simulink model "Simulation_03"  (R2014a)
settings: Solver=ode45  SolverMode=SingleTasking  StartTime=0.0  StopTime=5  FixedStep=1e-6  RelTol=1e-3
undefined symbols (not defined in the file or in its folder): sigbuilder_block
libraries: powerlib x12, simulink x2, powerlib_meascontrol x1
settings Model: CovModelRefEnable=off  Creator=Sunil Yaduvanshi  LastModifiedBy=Dell
settings SolverCC: AutoInsertRateTranBlk=on
settings DataIOCC: LimitDataPoints=off  SaveFormat=StructureWithTime
settings DebuggingCC: MergeDetectMultiDrivingBlocksExec=error  SolverPrmCheckMsg=none  FrameProcessingCompatibilityMsg=error
settings HardwareCC: ProdBitPerPointer=64  ProdLargestAtomicFloat=Float  ProdIntDivRoundTo=Zero  ProdEndianess=LittleEndian  ProdHWDeviceType=Specified
settings ModelReferenceCC: PropagateSignalLabelsOutOfModel=on

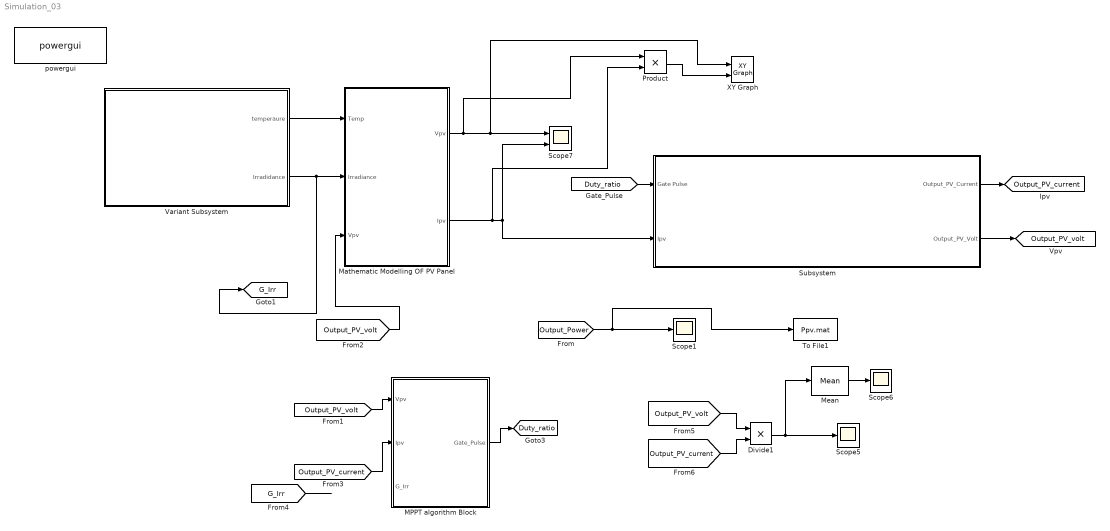
== system Simulation_03 ==
  Divide1 : Product  Inputs=**
  MPPT algorithm Block : Subsystem
  Mathematic Modelling OF PV Panel : Subsystem
      mask Display:
      | plot([0.3 0.4],[0.4 0.8]);
      | plot([0.4 0.5],[0.4 0.8]);
      | plot([0.5 0.6],[0.4 0.8]);
      | plot([0.6 0.7],[0.4 0.8]);
      | plot([0.3 0.6],[0.4 0.4]);
      | plot([0.325 0.625],[0.5 0.5]);
      | plot([0.35 0.65],[0.6 0.6]);
      | plot([0.375 0.675],[0.7 0.7]);
      | plot([0.4 0.7],[0.8 0.8]);
      | text(0.52,0.75,'PV module (V)','horizontalAlignment', 'center');
  Mean : powerlib_meascontrol/Measurements/Mean  Freq=60  Vinit=0  Ts=0
  Product : Product
  Scope1 : Scope
      settings: TimeRange=2  YMin=249.7  YMax=251.7  SaveName=ScopeData2
  Scope5 : Scope
      settings: TimeRange=0.8  YMin=222.5  YMax=262.5  SaveName=ScopeData6
  Scope6 : Scope
      settings: TimeRange=0.8  YMin=258.52  YMax=258.65  SaveName=ScopeData7
  Scope7 : Scope  NumInputPorts=2
      settings: YMin=34.5~6.825  YMax=37.5~7.275
  Subsystem : Subsystem
  To File1 : ToFile  Filename=Ppv.mat  SaveFormat=Timeseries
  Variant Subsystem : Subsystem  Variant=on
  XY Graph : simulink/Sinks/XY Graph  xmin=0  xmax=45  ymin=0  ymax=260  st=-1
  powergui : powerlib/powergui  Priority=1  SimulationMode=Discrete  SolverType=Tustin  SampleTime=1e-6  frequency=60  SPID=off  DisableSnubberDevices=off  DisableRonSwitches=off  DisableVfSwitches=off  SwTol=0  Interpol=off  DisplayEquations=off  Ts=0  methode=off  frequencyindice=0  Pbase=100e6  ErrMax=1e-4  Iterations=50  UnitsV=kV  UnitsW=MW  FunctionMessages=off  echomessages=off  HookPort=off  EnableUseOfTLC=off  x0status=blocks  RestoreLinks=warning  ResistiveCurrentMeasurement=off  Frange=[0:2:500]  Ylog=off  Xlog=on  ShowGrid=off  save=off  variable=ZData  structure=0  ZoomFFT=off  StartTime=0.0  cycles=1  DisplayStyle=1  fundamental=60  FreqAxis=off  MaxFrequency=1000  frequencyindicesteady=1  RmsSteady=1  display=off
  tag scope: Duty_ratio=global, G_Irr=global, Output_PV_current=global, Output_PV_volt=global
  wires:
  [Output_Power] -> To File1/1, Scope1/1
  [Output_PV_volt] -> Divide1/1
  [Output_PV_current] -> Divide1/2
  Divide1/1 -> Scope5/1, Mean/1
  Mean/1 -> Scope6/1
  Variant Subsystem/1(temperaure) -> Mathematic Modelling OF PV Panel/1(Temp)
  Variant Subsystem/2("Irradidance ") -> [G_Irr], Mathematic Modelling OF PV Panel/2(Irradiance)
  Mathematic Modelling OF PV Panel/2(Ipv) -> Product/2, Subsystem/2(Ipv), Scope7/2
  [Output_PV_volt] -> Mathematic Modelling OF PV Panel/3(Vpv)
  [Duty_ratio] -> Subsystem/1(Gate Pulse)
  Subsystem/1(Output_PV_Current) -> [Output_PV_current]
  Subsystem/2(Output_PV_Volt) -> [Output_PV_volt]
  [Output_PV_volt] -> MPPT algorithm Block/1(Vpv)
  [Output_PV_current] -> MPPT algorithm Block/2(Ipv)
  MPPT algorithm Block/1("Gate_Pulse ") -> [Duty_ratio]
  [G_Irr] -> ?
  Mathematic Modelling OF PV Panel/1("Vpv ") -> Product/1, XY Graph/1, Scope7/1
  Product/1 -> XY Graph/2

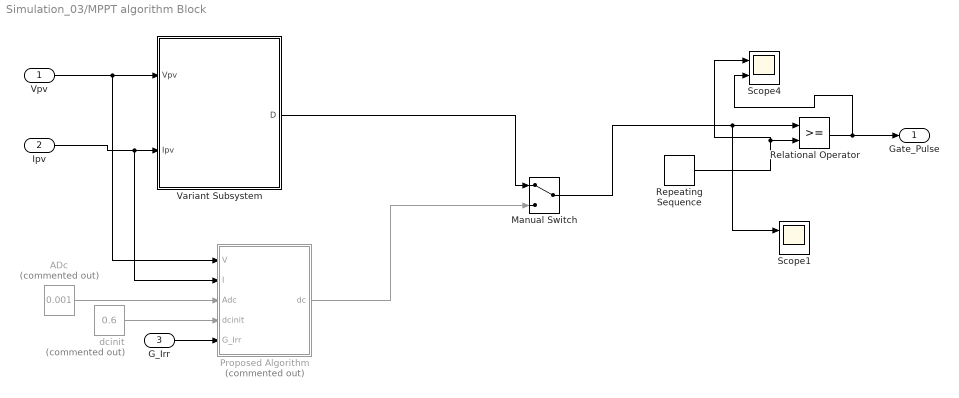
== system Simulation_03/MPPT algorithm Block ==
  Vpv : Inport
  Ipv : Inport  Port=2
  G_Irr : Inport  Port=3
  "ADc\t" : Constant  Commented=on  Value=0.001
  Manual Switch : ManualSwitch
  Proposed Algorithm : MATLAB Function  Commented=on  TreatAsAtomicUnit=on
  Relational Operator : RelationalOperator  OutDataTypeStr=boolean
  Repeating Sequence : simulink/Sources/Repeating Sequence  rep_seq_t=[0 1/40000 1/20000]  rep_seq_y=[0 1 0]
  Scope1 : Scope  NumInputPorts=2
      settings: YMin=2.6~0  YMax=2.9~1
  Scope4 : Scope  NumInputPorts=2
      settings: YMin=0~0  YMax=1~1  SaveName=ScopeData5
  Variant Subsystem : Subsystem  Variant=on
  dcinit : Constant  Commented=on  Value=0.6
  "Gate_Pulse " : Outport
  wires:
  Relational Operator/1 -> "Gate_Pulse "/1, Scope4/2
  Repeating Sequence/1 -> Scope4/1, Relational Operator/2
  Ipv/1 -> Proposed Algorithm/2(I), Variant Subsystem/2(Ipv)
  Vpv/1 -> Proposed Algorithm/1(V), Variant Subsystem/1(Vpv)
  Manual Switch/1 -> Scope1/1, Relational Operator/1
  Variant Subsystem/1(D) -> Manual Switch/1
  dcinit/1 -> Proposed Algorithm/4(dcinit)
  "ADc\t"/1 -> Proposed Algorithm/3(Adc)
  Proposed Algorithm/1(dc) -> Manual Switch/2
  G_Irr/1 -> Proposed Algorithm/5(G_Irr)

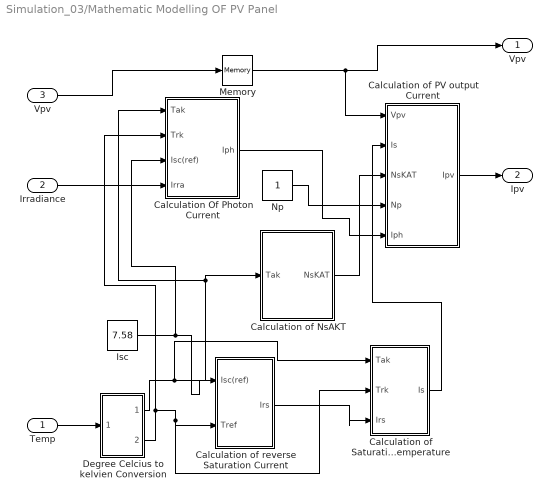
== system Simulation_03/Mathematic Modelling OF PV Panel ==
  Temp : Inport
  Irradiance : Inport  Port=2
  Vpv : Inport  Port=3
  "Calculation Of Photon Current " : Subsystem
  Calculation of Saturation Current Varies With Temperature : Subsystem
  Calculation of NsAKT : Subsystem
  "Calculation of PV output Current " : Subsystem
  Calculation of reverse Saturation Current : Subsystem
  Degree Celcius to kelvien Conversion : Subsystem
  Isc : Constant  Value=7.58
  Memory : Memory
  Np : Constant
  "Vpv " : Outport
  Ipv : Outport  Port=2
  wires:
  Calculation of Saturation Current Varies With Temperature/1(Is) -> "Calculation of PV output Current "/2(Is)
  Calculation of reverse Saturation Current/1(Irs) -> Calculation of Saturation Current Varies With Temperature/3("Irs ")
  Np/1 -> "Calculation of PV output Current "/4(Np)
  Temp/1 -> Degree Celcius to kelvien Conversion/1("Top ")
  "Calculation of PV output Current "/1("Ipv ") -> Ipv/1
  Irradiance/1 -> "Calculation Of Photon Current "/4(Irra)
  Degree Celcius to kelvien Conversion/1(Tak) -> Calculation of Saturation Current Varies With Temperature/1(Tak), "Calculation Of Photon Current "/1(Tak), Calculation of NsAKT/1("Tak ")
  "Calculation Of Photon Current "/1(Iph) -> "Calculation of PV output Current "/5(Iph)
  Calculation of NsAKT/1(NsKAT) -> "Calculation of PV output Current "/3(NsKAT)
  Isc/1 -> "Calculation Of Photon Current "/3(Isc(ref)), Calculation of reverse Saturation Current/1("Isc(ref) ")
  Degree Celcius to kelvien Conversion/2(Trk) -> "Calculation Of Photon Current "/2(Trk), Calculation of Saturation Current Varies With Temperature/2("Trk "), Calculation of reverse Saturation Current/2("Tref ")
  Vpv/1 -> Memory/1
  Memory/1 -> "Calculation of PV output Current "/1(Vpv), "Vpv "/1

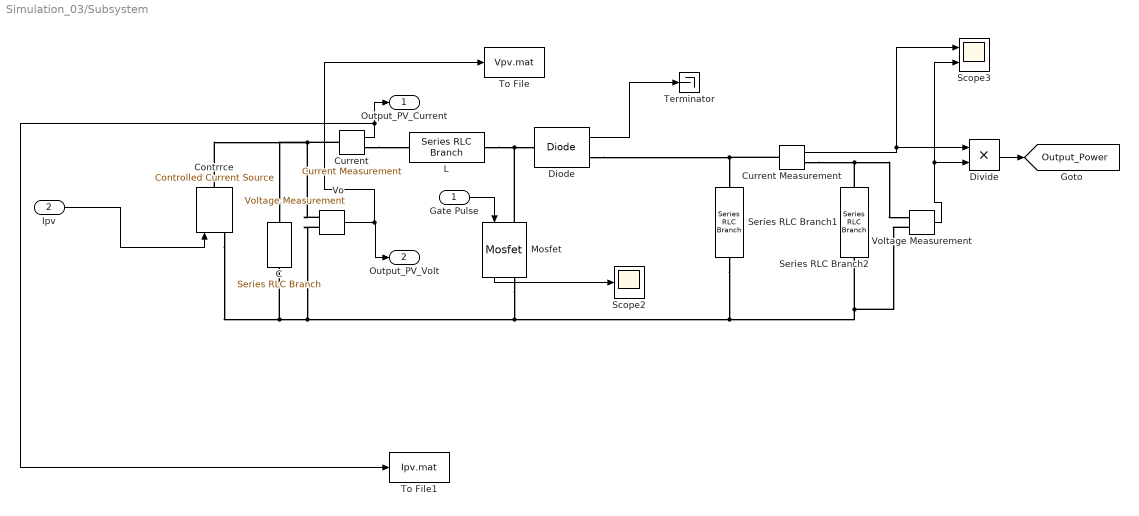
== system Simulation_03/Subsystem ==
  Gate Pulse : Inport
  Ipv : Inport  Port=2
  C : powerlib/Elements/Series RLC Branch  LConnTagsString=__new0  RConnTagsString=__new0  BranchType=C  Resistance=10  Inductance=5e-3  SetiL0=on  InitialCurrent=0  Capacitance=1e-6  Setx0=off  InitialVoltage=0  Measurements=None
  Contrrce : powerlib/Electrical Sources/Controlled Current Source  Initialize=on  Source_Type=DC  Amplitude=0  Phase=0  Frequency=0  Measurements=None
  "Current " : powerlib/Measurements/Current Measurement  PhasorSimulation=off  OutputType=Complex  PSBequivalent=0
  Current Measurement : powerlib/Measurements/Current Measurement  PhasorSimulation=off  OutputType=Complex  PSBequivalent=0
  Diode : powerlib/Power Electronics/Diode  Ron=0.001  Lon=0  Vf=0.8  IC=0  UseSnubber=off  Rs=500*0  Cs=250e-9*0  Measurements=on
  Divide : Product  Inputs=**
  L : powerlib/Elements/Series RLC Branch  LConnTagsString=__new0  RConnTagsString=__new0  BranchType=L  Resistance=10  Inductance=5e-3  SetiL0=on  InitialCurrent=0  Capacitance=1e-6  Setx0=off  InitialVoltage=0  Measurements=None
  Mosfet : powerlib/Power Electronics/Mosfet  Ron=0.1  Lon=0  Rd=0.01  Vfd=0  IC=0  Rs=1e5  Cs=inf  Measurements=on
  Scope2 : Scope
      settings: YMin=-5.49725  YMax=49.47525  SaveName=ScopeData3
  Scope3 : Scope  NumInputPorts=2
      settings: YMin=2.52~100.8  YMax=2.536~101.45  SaveName=ScopeData4
  Series RLC Branch1 : powerlib/Elements/Series RLC Branch  LConnTagsString=__new0  RConnTagsString=__new0  BranchType=C  Resistance=1  Inductance=5e-3  SetiL0=on  InitialCurrent=0  Capacitance=270e-6  Setx0=on  InitialVoltage=0  Measurements=None
  Series RLC Branch2 : powerlib/Elements/Series RLC Branch  LConnTagsString=__new0  RConnTagsString=__new0  BranchType=R  Resistance=60  Inductance=5e-3  SetiL0=on  InitialCurrent=0  Capacitance=1e-6  Setx0=off  InitialVoltage=0  Measurements=None
  Terminator : Terminator
  To File : ToFile  Filename=Vpv.mat  SaveFormat=Timeseries
  To File1 : ToFile  Filename=Ipv.mat  SaveFormat=Timeseries
  Vo : powerlib/Measurements/Voltage Measurement  PhasorSimulation=off  OutputType=Complex  PSBequivalent=0
  Voltage Measurement : powerlib/Measurements/Voltage Measurement  PhasorSimulation=off  OutputType=Complex  PSBequivalent=0
  Output_PV_Current : Outport
  Output_PV_Volt : Outport  Port=2
  tag scope: Output_Power=global
  wires:
  Ipv/1 -> Contrrce/1
  Diode/1 -> Terminator/1
  Divide/1 -> [Output_Power]
  Voltage Measurement/1 -> Scope3/2, Divide/2
  Vo/1 -> To File/1, Output_PV_Volt/1
  Gate Pulse/1 -> Mosfet/1
  "Current "/1 -> To File1/1, Output_PV_Current/1
  Current Measurement/1 -> Divide/1, Scope3/1
  Mosfet/1 -> Scope2/1
  connections:
  Diode/RConn1 -- Current Measurement/LConn1 -- Series RLC Branch1/LConn1
  Vo/LConn1 -- Contrrce/RConn1 -- C/LConn1 -- "Current "/LConn1
  Series RLC Branch2/LConn1 -- Current Measurement/RConn1 -- Voltage Measurement/LConn1
  Contrrce/LConn1 -- C/RConn1 -- Vo/LConn2 -- Mosfet/RConn1 -- Series RLC Branch1/RConn1 -- Voltage Measurement/LConn2 -- Series RLC Branch2/RConn1
  "Current "/RConn1 -- L/LConn1
  L/RConn1 -- Mosfet/LConn1 -- Diode/LConn1

== system Simulation_03/Variant Subsystem ==
  note: 1) Only subsystems can be added as variant choices at this level
      | 2) Blocks cannot be connected at this level as connectivity is
      | automatically determined at simulation, based on the active variant
  Irradiance Variatioin : Subsystem  TreatAsAtomicUnit=on  VariantControl=Irradiance
  "Temperature Variation " : Subsystem  TreatAsAtomicUnit=on  VariantControl=Temperature
  temperaure : Outport
  "Irradidance " : Outport  Port=2

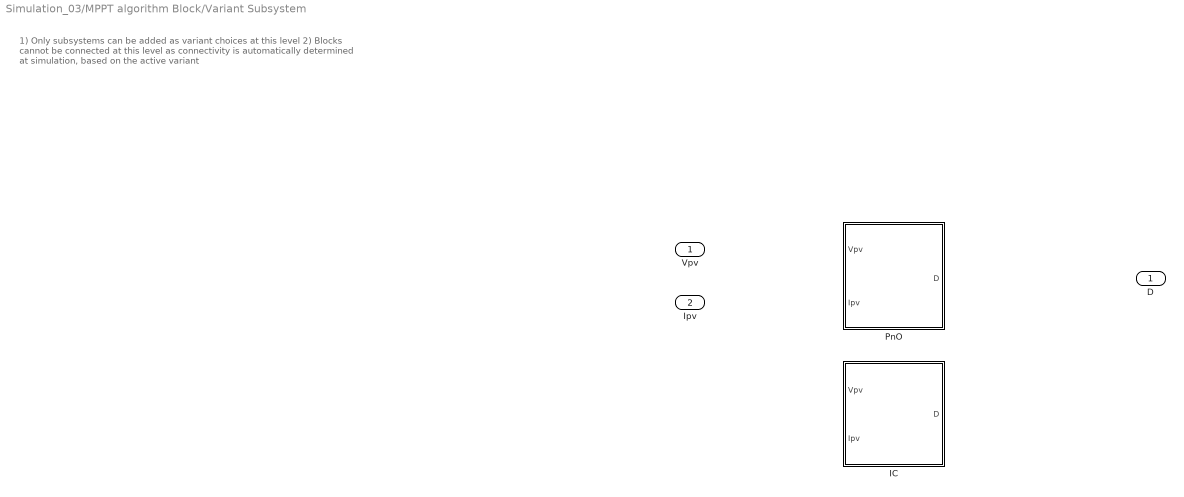
== system Simulation_03/MPPT algorithm Block/Variant Subsystem ==
  note: 1) Only subsystems can be added as variant choices at this level
      | 2) Blocks cannot be connected at this level as connectivity is
      | automatically determined at simulation, based on the active variant
  Vpv : Inport
  Ipv : Inport  Port=2
  IC : Subsystem  TreatAsAtomicUnit=on  VariantControl=IC
  PnO : Subsystem  TreatAsAtomicUnit=on  VariantControl=PnO
  D : Outport

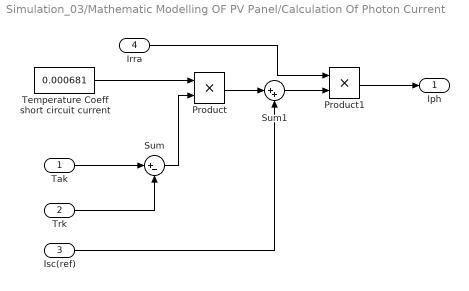
== system Simulation_03/Mathematic Modelling OF PV Panel/Calculation Of Photon Current  ==
  Tak : Inport
  Trk : Inport  Port=2
  Isc(ref) : Inport  Port=3
  Irra : Inport  Port=4
  Product : Product
  Product1 : Product
  Sum : Sum  Inputs=|+-
  Sum1 : Sum  Inputs=|++
  "Temperature Coeff short circuit current " : Constant  Value=0.000681
  Iph : Outport
  wires:
  Product/1 -> Sum1/1
  Trk/1 -> Sum/2
  "Temperature Coeff short circuit current "/1 -> Product/1
  Irra/1 -> Product1/1
  Isc(ref)/1 -> Sum1/2
  Tak/1 -> Sum/1
  Sum1/1 -> Product1/2
  Sum/1 -> Product/2
  Product1/1 -> Iph/1

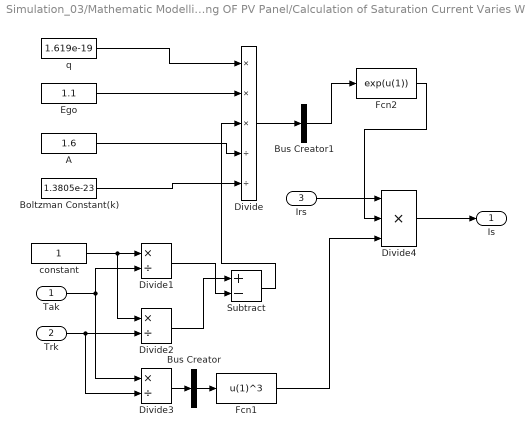
== system Simulation_03/Mathematic Modelling OF PV Panel/Calculation of Saturation Current Varies With Temperature ==
  Tak : Inport
  "Trk " : Inport  Port=2
  "Irs " : Inport  Port=3
  "A " : Constant  Value=1.6
  Boltzman Constant(k) : Constant  Value=1.3805e-23
  Bus Creator : BusCreator  Inputs=1
  Bus Creator1 : BusCreator  Inputs=1
  Divide : Product  Inputs=***//
  Divide1 : Product  Inputs=*/
  Divide2 : Product  Inputs=*/
  Divide3 : Product  Inputs=*/
  Divide4 : Product  Inputs=***
  Ego : Constant  Value=1.1
  Fcn1 : Fcn  Expr=u(1)^3
  Fcn2 : Fcn  Expr=exp(u(1))
  Subtract : Sum  Inputs=+-
  "constant " : Constant
  "q " : Constant  Value=1.619e-19
  Is : Outport
  wires:
  "constant "/1 -> Divide2/1, Divide1/1
  Bus Creator1/1 -> Fcn2/1
  Divide/1 -> Bus Creator1/1
  Divide1/1 -> Subtract/2
  Fcn1/1 -> Divide4/3
  Divide2/1 -> Subtract/1
  Tak/1 -> Divide1/2, Divide3/1
  Fcn2/1 -> Divide4/2
  "Trk "/1 -> Divide3/2, Divide2/2
  "A "/1 -> Divide/4
  Ego/1 -> Divide/2
  Subtract/1 -> Divide/3
  Boltzman Constant(k)/1 -> Divide/5
  "q "/1 -> Divide/1
  "Irs "/1 -> Divide4/1
  Divide4/1 -> Is/1
  Bus Creator/1 -> Fcn1/1
  Divide3/1 -> Bus Creator/1

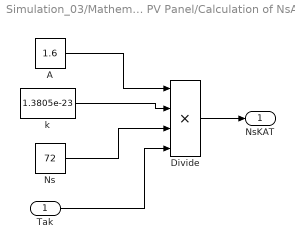
== system Simulation_03/Mathematic Modelling OF PV Panel/Calculation of NsAKT ==
  "Tak " : Inport
  A : Constant  Value=1.6
  Divide : Product  Inputs=****
  Ns : Constant  Value=72
  k : Constant  Value=1.3805e-23
  NsKAT : Outport
  wires:
  Ns/1 -> Divide/3
  A/1 -> Divide/1
  k/1 -> Divide/2
  "Tak "/1 -> Divide/4
  Divide/1 -> NsKAT/1

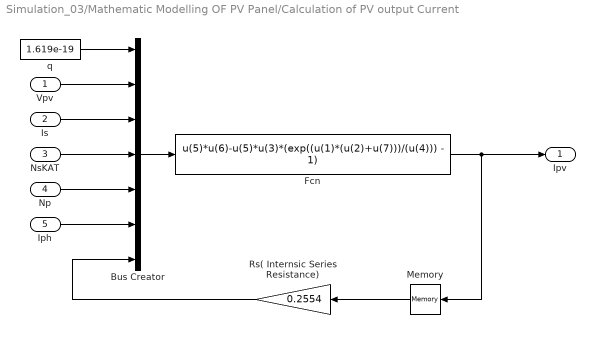
== system Simulation_03/Mathematic Modelling OF PV Panel/Calculation of PV output Current  ==
  Vpv : Inport
  Is : Inport  Port=2
  NsKAT : Inport  Port=3
  Np : Inport  Port=4
  Iph : Inport  Port=5
  Bus Creator : BusCreator  Inputs=7
  Fcn : Fcn  Expr=u(5)*u(6)-u(5)*u(3)*(exp((u(1)*(u(2)+u(7)))/(u(4))) - 1)
  Memory : Memory
  Rs( Internsic Series Resistance) : Gain  Gain=0.2554
  q : Constant  Value=1.619e-19
  "Ipv " : Outport
  wires:
  Vpv/1 -> Bus Creator/2
  Is/1 -> Bus Creator/3
  Fcn/1 -> Memory/1, "Ipv "/1
  Bus Creator/1 -> Fcn/1
  Rs( Internsic Series Resistance)/1 -> Bus Creator/7
  Iph/1 -> Bus Creator/6
  Np/1 -> Bus Creator/5
  q/1 -> Bus Creator/1
  NsKAT/1 -> Bus Creator/4
  Memory/1 -> Rs( Internsic Series Resistance)/1

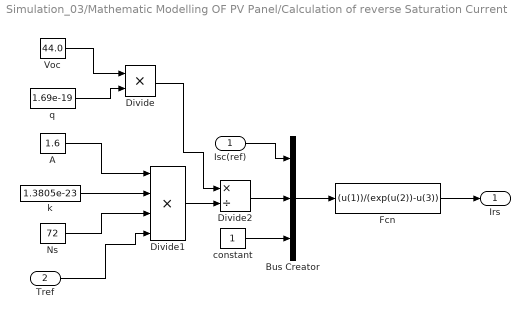
== system Simulation_03/Mathematic Modelling OF PV Panel/Calculation of reverse Saturation Current ==
  "Isc(ref) " : Inport
  "Tref " : Inport  Port=2
  A : Constant  Value=1.6
  Bus Creator : BusCreator  Inputs=3
  Divide : Product  Inputs=**
  Divide1 : Product  Inputs=****
  Divide2 : Product  Inputs=*/
  Fcn : Fcn  Expr=(u(1))/(exp(u(2))-u(3))
  Ns : Constant  Value=72
  Voc : Constant  Value=44.0
  "constant " : Constant
  k : Constant  Value=1.3805e-23
  q : Constant  Value=1.69e-19
  Irs : Outport
  wires:
  Voc/1 -> Divide/1
  Divide/1 -> Divide2/1
  k/1 -> Divide1/2
  "constant "/1 -> Bus Creator/3
  Divide2/1 -> Bus Creator/2
  Bus Creator/1 -> Fcn/1
  "Tref "/1 -> Divide1/4
  Fcn/1 -> Irs/1
  q/1 -> Divide/2
  A/1 -> Divide1/1
  "Isc(ref) "/1 -> Bus Creator/1
  Ns/1 -> Divide1/3
  Divide1/1 -> Divide2/2

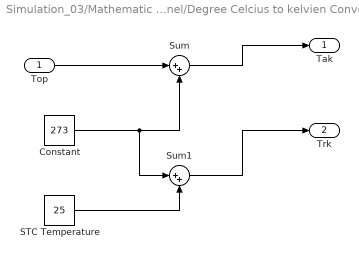
== system Simulation_03/Mathematic Modelling OF PV Panel/Degree Celcius to kelvien Conversion ==
  "Top " : Inport
  Constant : Constant  Value=273
  STC Temperature : Constant  Value=25
  Sum : Sum  Inputs=|++
  Sum1 : Sum  Inputs=|++
  Tak : Outport
  Trk : Outport  Port=2
  wires:
  Sum1/1 -> Trk/1
  Constant/1 -> Sum1/1, Sum/2
  "Top "/1 -> Sum/1
  Sum/1 -> Tak/1
  STC Temperature/1 -> Sum1/2

== system Simulation_03/Variant Subsystem/Irradiance Variatioin ==
  Insolation1 : Subsystem  Tag=STV Subsys  LoadFcn=sigbuilder_block('load');  StartFcn=sigbuilder_block('start');  StopFcn=sigbuilder_block('stop');  ClipboardFcn=sigbuilder_block('clipboard');  mask(Sigbuilder block){}
      mask help: Simulink:masks:SigbuilderBlock_MD
      mask init:
      | if ~strcmp(get_param(bdroot(gcbh),'SimulationStatus'),'stopped') tuvar = sigbuilder_block('maskInit'); end
      settings: CopyFcn=sigbuilder_block('copy');  DeleteFcn=sigbuilder_block('delete');  ModelCloseFcn=sigbuilder_block('modelClose');  PreSaveFcn=sigbuilder_block('preSave');  PauseFcn=sigbuilder_block('pause')  ContinueFcn=sigbuilder_block('continue')  NameChangeFcn=sigbuilder_block('namechange');  OpenFcn=sigbuilder_block('open',[211.5 118.5 550.5 394.5 ]);  CloseFcn=sigbuilder_block('close');
      mask Display: plot(0, 0, 100, 100,[2, 2, 32, 32, 2], [68, 8, 8, 68, 68],[32, 2], [38, 38], [32, 19, 2],[53, 60, 44], [32, 17, 17, 2],[16, 16, 31, 31]);txt = getActiveGroup(gcbh);text(2, 100, txt,'verticalAlignment', 'top');
  "Temperature " : Subsystem  Tag=STV Subsys  LoadFcn=sigbuilder_block('load');  StartFcn=sigbuilder_block('start');  StopFcn=sigbuilder_block('stop');  ClipboardFcn=sigbuilder_block('clipboard');  mask(Sigbuilder block){}
      mask help: Simulink:masks:SigbuilderBlock_MD
      mask init:
      | if ~strcmp(get_param(bdroot(gcbh),'SimulationStatus'),'stopped') tuvar = sigbuilder_block('maskInit'); end
      settings: CopyFcn=sigbuilder_block('copy');  DeleteFcn=sigbuilder_block('delete');  ModelCloseFcn=sigbuilder_block('modelClose');  PreSaveFcn=sigbuilder_block('preSave');  PauseFcn=sigbuilder_block('pause');  ContinueFcn=sigbuilder_block('continue');  NameChangeFcn=sigbuilder_block('namechange');  OpenFcn=sigbuilder_block('open',[351 -51.75 543 385.5 ]);  CloseFcn=sigbuilder_block('close');
      mask Display: plot(0, 0, 100, 100,[2, 2, 32, 32, 2], [68, 8, 8, 68, 68],[32, 2], [38, 38], [32, 19, 2],[53, 60, 44], [32, 17, 17, 2],[16, 16, 31, 31]);txt = getActiveGroup(gcbh);text(2, 100, txt,'verticalAlignment', 'top');
  temperaure : Outport
  "Irradidance " : Outport  Port=2
  wires:
  "Temperature "/1(Signal 1) -> temperaure/1
  Insolation1/1(irradiation) -> "Irradidance "/1

== system Simulation_03/Variant Subsystem/Temperature Variation  ==
  Insolation1 : Subsystem  Tag=STV Subsys  LoadFcn=sigbuilder_block('load');  StartFcn=sigbuilder_block('start');  StopFcn=sigbuilder_block('stop');  ClipboardFcn=sigbuilder_block('clipboard');  mask(Sigbuilder block){}
      mask help: Simulink:masks:SigbuilderBlock_MD
      mask init:
      | if ~strcmp(get_param(bdroot(gcbh),'SimulationStatus'),'stopped') tuvar = sigbuilder_block('maskInit'); end
      settings: CopyFcn=sigbuilder_block('copy');  DeleteFcn=sigbuilder_block('delete');  ModelCloseFcn=sigbuilder_block('modelClose');  PreSaveFcn=sigbuilder_block('preSave');  PauseFcn=sigbuilder_block('pause')  ContinueFcn=sigbuilder_block('continue')  NameChangeFcn=sigbuilder_block('namechange');  OpenFcn=sigbuilder_block('open',[557.25 17.25 550.5 394.5 ]);  CloseFcn=sigbuilder_block('close');
      mask Display: plot(0, 0, 100, 100,[2, 2, 32, 32, 2], [68, 8, 8, 68, 68],[32, 2], [38, 38], [32, 19, 2],[53, 60, 44], [32, 17, 17, 2],[16, 16, 31, 31]);txt = getActiveGroup(gcbh);text(2, 100, txt,'verticalAlignment', 'top');
  Temperature : Subsystem  Tag=STV Subsys  LoadFcn=sigbuilder_block('load');  StartFcn=sigbuilder_block('start');  StopFcn=sigbuilder_block('stop');  ClipboardFcn=sigbuilder_block('clipboard');  mask(Sigbuilder block){}
      mask help: Simulink:masks:SigbuilderBlock_MD
      mask init:
      | if ~strcmp(get_param(bdroot(gcbh),'SimulationStatus'),'stopped') tuvar = sigbuilder_block('maskInit'); end
      settings: CopyFcn=sigbuilder_block('copy');  DeleteFcn=sigbuilder_block('delete');  ModelCloseFcn=sigbuilder_block('modelClose');  PreSaveFcn=sigbuilder_block('preSave');  PauseFcn=sigbuilder_block('pause');  ContinueFcn=sigbuilder_block('continue');  NameChangeFcn=sigbuilder_block('namechange');  OpenFcn=sigbuilder_block('open',[437.25 180 550.5 395.25 ]);  CloseFcn=sigbuilder_block('close');
      mask Display: plot(0, 0, 100, 100,[2, 2, 32, 32, 2], [68, 8, 8, 68, 68],[32, 2], [38, 38], [32, 19, 2],[53, 60, 44], [32, 17, 17, 2],[16, 16, 31, 31]);txt = getActiveGroup(gcbh);text(2, 100, txt,'verticalAlignment', 'top');
  temperaure : Outport
  "Irradidance " : Outport  Port=2
  wires:
  Temperature/1(Signal 1) -> temperaure/1
  Insolation1/1(irradiation) -> "Irradidance "/1

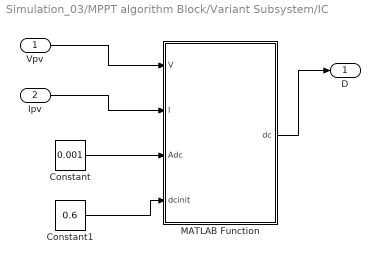
== system Simulation_03/MPPT algorithm Block/Variant Subsystem/IC ==
  Vpv : Inport  OutDataTypeStr=double  PortDimensions=1  SampleTime=[0.0001,0]
  Ipv : Inport  Port=2  OutDataTypeStr=double  PortDimensions=1  SampleTime=[0.0001,0]
  Constant : Constant  Value=0.001
  Constant1 : Constant  Value=0.6
  MATLAB Function : MATLAB Function  TreatAsAtomicUnit=on
  D : Outport  OutDataTypeStr=double  PortDimensions=1  SampleTime=[0.0001,0]
  wires:
  Vpv/1 -> MATLAB Function/1(V)
  Ipv/1 -> MATLAB Function/2(I)
  MATLAB Function/1(dc) -> D/1
  Constant1/1 -> MATLAB Function/4(dcinit)
  Constant/1 -> MATLAB Function/3(Adc)

== system Simulation_03/MPPT algorithm Block/Variant Subsystem/PnO ==
  Vpv : Inport
  Ipv : Inport  Port=2
  MATLAB Function : MATLAB Function  TreatAsAtomicUnit=on
  D : Outport
  wires:
  Ipv/1 -> MATLAB Function/2(PV_current)
  Vpv/1 -> MATLAB Function/1(PV_volt)
  MATLAB Function/1(D) -> D/1

== system Simulation_03/Variant Subsystem/Irradiance Variatioin/Insolation1 ==
  Demux : Demux  Tag=STV Demux  Outputs=1
  FromWs : FromWorkspace  Tag=STV FromWs  VariableName=tuvar  SampleTime=0
      SigBuilderData=|
      | common.afterFinalStr = 'Extrapolate'
      | common.sampleTime = 0
      | dataSet.timeRange = [0 6]
      | dataSet.name = 'Group 1'
      | sbobj.Groups.Name = 'Group 1'
      | sbobj.Groups.Signals.Name = 'irradiation'
      | sbobj.Groups.Signals.XData = [0 2 2 3.99 4 6]
      | sbobj.Groups.Signals.YData = [0.6 0.6 0.8 0.8 1 1]
  irradiation : Outport  Tag=STV Outport
  wires:
  FromWs/1 -> Demux/1
  Demux/1 -> irradiation/1

== system Simulation_03/Variant Subsystem/Irradiance Variatioin/Temperature  ==
  Demux : Demux  Tag=STV Demux  Outputs=1
  FromWs : FromWorkspace  Tag=STV FromWs  VariableName=tuvar  SampleTime=0
      SigBuilderData=|
      | common.afterFinalStr = 'Extrapolate'
      | common.sampleTime = 0
      | dataSet.timeRange = [0 10]
      | dataSet.name = 'Group 1'
      | sbobj.Groups.Name = 'Group 1'
      | sbobj.Groups.Signals.Name = 'Signal 1'
      | sbobj.Groups.Signals.XData = [0 1 2 10]
      | sbobj.Groups.Signals.YData = [25 25 25 25]
  Signal 1 : Outport  Tag=STV Outport
  wires:
  FromWs/1 -> Demux/1
  Demux/1 -> Signal 1/1

== system Simulation_03/Variant Subsystem/Temperature Variation /Insolation1 ==
  Demux : Demux  Tag=STV Demux  Outputs=1
  FromWs : FromWorkspace  Tag=STV FromWs  VariableName=tuvar  SampleTime=0
      SigBuilderData=|
      | common.afterFinalStr = 'Extrapolate'
      | common.sampleTime = 0
      | dataSet.timeRange = [0 6]
      | dataSet.name = 'Group 1'
      | sbobj.Groups.Name = 'Group 1'
      | sbobj.Groups.Signals.Name = 'irradiation'
      | sbobj.Groups.Signals.XData = [0 2 3.99 4 6]
      | sbobj.Groups.Signals.YData = [1 1 1 1 1]
  irradiation : Outport  Tag=STV Outport
  wires:
  FromWs/1 -> Demux/1
  Demux/1 -> irradiation/1

== system Simulation_03/Variant Subsystem/Temperature Variation /Temperature ==
  Demux : Demux  Tag=STV Demux  Outputs=1
  FromWs : FromWorkspace  Tag=STV FromWs  VariableName=tuvar  SampleTime=0
      SigBuilderData=|
      | common.afterFinalStr = 'Extrapolate'
      | common.sampleTime = 0
      | dataSet.timeRange = [0 10]
      | dataSet.name = 'Group 1'
      | sbobj.Groups.Name = 'Group 1'
      | sbobj.Groups.Signals.Name = 'Signal 1'
      | sbobj.Groups.Signals.XData = [0 2 4 10]
      | sbobj.Groups.Signals.YData = [25 25 25 25]
  Signal 1 : Outport  Tag=STV Outport
  wires:
  Demux/1 -> Signal 1/1
  FromWs/1 -> Demux/1

== matlab function Simulation_03/MPPT algorithm Block/Variant Subsystem/IC/MATLAB Function ==
  data: V input; dc output; I input; Adc input; dcinit input
function dc = IC( V, I, Adc, dcinit)


persistent dco Vold Iold
dataType = 'double';

if isempty(Vold)
    Vold=0;
    Iold=0;
    dco=dcinit;
end


dV=V-Vold;
dI=I-Iold;

if dV==0
    if dI==0
        dc =dco;
        return
    else
        if dI>0
            dc = dco + Adc; 
        else
            dc = dco - Adc; 
        end
    end
else
    if I+(dI/dV)*V==0
        dc=dco;
        return
    else
        if I+(dI/dV)*V>0
            dc = dco - Adc; 
        else
            dc = dco + Adc; 
        end
    end
end
dcmax=0.95; 
  dcmin=0.05;
if dc>=dcmax || dc<=dcmin
    dc=dco;
end

dco=dc;
Vold=V;
Iold=I;
end

== matlab function Simulation_03/MPPT algorithm Block/Variant Subsystem/PnO/MATLAB Function ==
  data: PV_volt input; D output; PV_current input
function D   = fcn(PV_volt,PV_current)
%#codegen
persistent V1 I1 V0 I0 D0 

if isempty(D0)
V0 = 0;
I0 = 0;
D0 = 0.60;
end


P0 = V0*I0;
V1 = PV_volt;
I1 = PV_current;
P1=V1*I1;

if(P1>=P0)
    if(V1>=V0)
        D0=D0-0.001;
    else
        D0=D0+0.001;
    end
end
if(P1<P0)
    if(V1>=V0)
        D0=D0+0.001;
    else
        D0=D0-0.001;
    end
end
D=D0;
V0=V1;
I0=I1;



end

== matlab function Simulation_03/MPPT algorithm Block/Proposed Algorithm ==
  data: V input; dc output; I input; Adc input; dcinit input; G_Irr input
function dc = IC( V, I, Adc, dcinit, G_Irr)


persistent dco Vo Io
dataType = 'double';
   
            if isempty(Vo)
                Vo=0;
                Io=0;
                dco=dcinit;
            end

          
            dV=V-Vo;
            dI=I-Io;
          
            if dV==0
                if dI==0
                    dc =dco;
                    return
                else
                    if dI>0
                        dc = dco + Adc; 
                    else
                        dc = dco - Adc; 
                    end
                end
            else
                if I+(dI/dV)*V==0
                    dc=dco;
                    return
                else
                    if I+(dI/dV)*V>0
                        dc = dco - Adc; 
                    else
                        dc = dco + Adc; 
                    end
                end
            end
            dcmax=0.95; 
              dcmin=0.05;
            if dc>=dcmax || dc<=dcmin
                dc=dco;
            end

            dco=dc;
            Vo=V;
            Io=I;
     
         
     end
